simulink model "Quadrotor_two_blocks_v3"  (R2020a)
settings: Solver=FixedStepAuto  StartTime=0.0  StopTime=options.T_train  FixedStep=options.dt  RelTol=1e-6
undefined symbols (not defined in the file or in its folder): options, Quad
libraries: neural x87
(part 3 of 5)

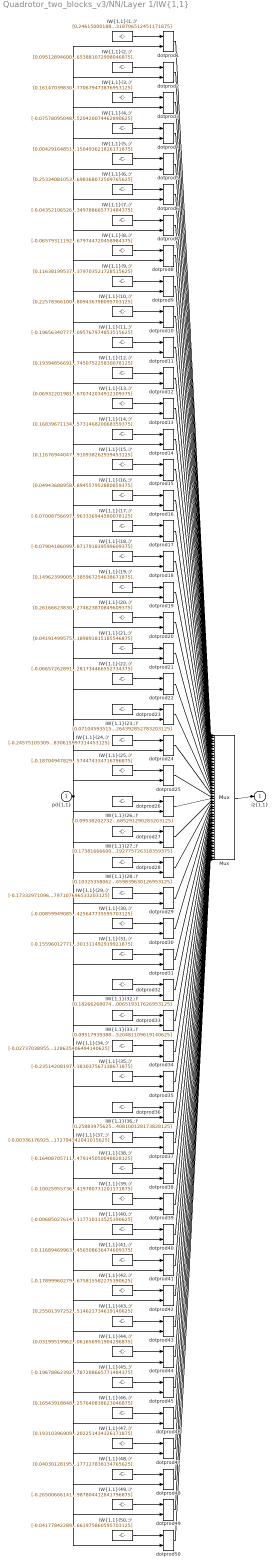
== system Quadrotor_two_blocks_v3/NN/Layer 1/IW{1,1} ==
  "pd{1,1}" : Inport  PortDimensions=15
      mask Display: e = 0.06;c1 = [120 230 180]/255;c2 = ([120 230 180]+0)/(256+128);c3 = ([120 230 180]+128)/(256+128);patch([0 1 1 0],[0 0 1 1],c1);patch([0 1 1 1-e 1-e 0+e],[0 0 1 1-e 0+e 0+e],c2);patch([0 0 1 1-e 0+e 0+e],[0 1 1 1-e 1-e 0+e],c3);plot([0 1 1 0 0],[0 0 1 1 0]);
  "IW{1,1}(1,:)'" : Constant  Value=[0.24615000188350677490234375;-0.2769688665866851806640625;0.19857059419155120849609375;-0.188253819942474365234375;-0.2332561910152435302734375;0.2510521709918975830078125;0.09584285318851470947265625;0.19580931961536407470703125;-0.05497033894062042236328125;-0.1999491155147552490234375;0.0023749410174787044525146484375;-0.1995990574359893798828125;-0.03645892441272735595703125;0.22868992388248443603515625;0.1527912318706512451171875]
      mask Display: e = 0.06;c1 = [120 150 230]/255;c2 = ([120 150 230]+0)/383;c3 = ([120 150 230]+128)/383;patch([0 1 1 0],[0 0 1 1],c1);patch([0 1 1 1-e 1-e 0+e],[0 0 1 1-e 0+e 0+e],c2);patch([0 0 1 1-e 0+e 0+e],[0 1 1 1-e 1-e 0+e],c3);plot([0 1 1 0 0],[0 0 1 1 0]);disp('Weights');
  "IW{1,1}(10,:)'" : Constant  Value=[0.22578366100788116455078125;0.1848590075969696044921875;0.02715091407299041748046875;-0.2515232563018798828125;-0.119150958955287933349609375;-0.2643735110759735107421875;-0.170074880123138427734375;-0.12265492975711822509765625;-0.15844647586345672607421875;-0.035431392490863800048828125;-0.012248366139829158782958984375;0.2504398822784423828125;0.2176316678524017333984375;-0.121464140713214874267578125;0.24602694809436798095703125]
      mask Display: e = 0.06;c1 = [120 150 230]/255;c2 = ([120 150 230]+0)/383;c3 = ([120 150 230]+128)/383;patch([0 1 1 0],[0 0 1 1],c1);patch([0 1 1 1-e 1-e 0+e],[0 0 1 1-e 0+e 0+e],c2);patch([0 0 1 1-e 0+e 0+e],[0 1 1 1-e 1-e 0+e],c3);plot([0 1 1 0 0],[0 0 1 1 0]);disp('Weights');
  "IW{1,1}(11,:)'" : Constant  Value=[-0.19656340777873992919921875;0.19387482106685638427734375;-0.0459356568753719329833984375;0.2647550404071807861328125;0.2745810449123382568359375;0.041675679385662078857421875;0.12391470372676849365234375;-0.16976629197597503662109375;0.0317076109349727630615234375;0.080004759132862091064453125;0.18198011815547943115234375;0.2869862020015716552734375;-0.145103871822357177734375;-0.1056883335113525390625;-0.17829205095767974853515625]
      mask Display: e = 0.06;c1 = [120 150 230]/255;c2 = ([120 150 230]+0)/383;c3 = ([120 150 230]+128)/383;patch([0 1 1 0],[0 0 1 1],c1);patch([0 1 1 1-e 1-e 0+e],[0 0 1 1-e 0+e 0+e],c2);patch([0 0 1 1-e 0+e 0+e],[0 1 1 1-e 1-e 0+e],c3);plot([0 1 1 0 0],[0 0 1 1 0]);disp('Weights');
  "IW{1,1}(12,:)'" : Constant  Value=[0.193948566913604736328125;-0.19000457227230072021484375;-0.086530886590480804443359375;-0.180632650852203369140625;-0.19515524804592132568359375;-0.0314301587641239166259765625;0.1326048672199249267578125;0.2292857468128204345703125;0.13057291507720947265625;-0.196017682552337646484375;-0.267640650272369384765625;0.018295593559741973876953125;0.092189691960811614990234375;0.2637727260589599609375;0.3198082745075225830078125]
      mask Display: e = 0.06;c1 = [120 150 230]/255;c2 = ([120 150 230]+0)/383;c3 = ([120 150 230]+128)/383;patch([0 1 1 0],[0 0 1 1],c1);patch([0 1 1 1-e 1-e 0+e],[0 0 1 1-e 0+e 0+e],c2);patch([0 0 1 1-e 0+e 0+e],[0 1 1 1-e 1-e 0+e],c3);plot([0 1 1 0 0],[0 0 1 1 0]);disp('Weights');
  "IW{1,1}(13,:)'" : Constant  Value=[0.0693220198154449462890625;-0.2461332976818084716796875;-0.0500579774379730224609375;0.154254257678985595703125;0.03849256038665771484375;0.23319505155086517333984375;-0.2198602855205535888671875;0.0940903127193450927734375;0.068703256547451019287109375;0.3237433731555938720703125;0.282208859920501708984375;0.054376460611820220947265625;-0.110324062407016754150390625;-0.195249617099761962890625;0.1259351670742034912109375]
      mask Display: e = 0.06;c1 = [120 150 230]/255;c2 = ([120 150 230]+0)/383;c3 = ([120 150 230]+128)/383;patch([0 1 1 0],[0 0 1 1],c1);patch([0 1 1 1-e 1-e 0+e],[0 0 1 1-e 0+e 0+e],c2);patch([0 0 1 1-e 0+e 0+e],[0 1 1 1-e 1-e 0+e],c3);plot([0 1 1 0 0],[0 0 1 1 0]);disp('Weights');
  "IW{1,1}(14,:)'" : Constant  Value=[0.1683967113494873046875;-0.20133976638317108154296875;-0.0863095223903656005859375;-0.20713274180889129638671875;-0.0525672137737274169921875;0.090336024761199951171875;0.209331095218658447265625;-0.02543685026466846466064453125;-0.2690856456756591796875;-0.12498508393764495849609375;-0.2766831815242767333984375;-0.08764405548572540283203125;-0.082091726362705230712890625;0.0041847997345030307769775390625;0.035477362573146820068359375]
      mask Display: e = 0.06;c1 = [120 150 230]/255;c2 = ([120 150 230]+0)/383;c3 = ([120 150 230]+128)/383;patch([0 1 1 0],[0 0 1 1],c1);patch([0 1 1 1-e 1-e 0+e],[0 0 1 1-e 0+e 0+e],c2);patch([0 0 1 1-e 0+e 0+e],[0 1 1 1-e 1-e 0+e],c3);plot([0 1 1 0 0],[0 0 1 1 0]);disp('Weights');
  "IW{1,1}(15,:)'" : Constant  Value=[0.116769440472126007080078125;0.1042247116565704345703125;0.237415611743927001953125;-0.2428454458713531494140625;0.040846385061740875244140625;-0.13717560470104217529296875;0.063017547130584716796875;-0.13246162235736846923828125;0.262563228607177734375;-0.05162282288074493408203125;-0.076942525804042816162109375;0.0027029174380004405975341796875;-0.069335155189037322998046875;0.075416088104248046875;-0.17622537910938262939453125]
      mask Display: e = 0.06;c1 = [120 150 230]/255;c2 = ([120 150 230]+0)/383;c3 = ([120 150 230]+128)/383;patch([0 1 1 0],[0 0 1 1],c1);patch([0 1 1 1-e 1-e 0+e],[0 0 1 1-e 0+e 0+e],c2);patch([0 0 1 1-e 0+e 0+e],[0 1 1 1-e 1-e 0+e],c3);plot([0 1 1 0 0],[0 0 1 1 0]);disp('Weights');
  "IW{1,1}(16,:)'" : Constant  Value=[0.049436889588832855224609375;0.21147786080837249755859375;-0.14443112909793853759765625;0.014394345693290233612060546875;-0.1196068823337554931640625;0.19549985229969024658203125;0.0031798514537513256072998046875;0.116258658468723297119140625;0.01721403189003467559814453125;-0.01672693900763988494873046875;0.107975371181964874267578125;-0.1965630948543548583984375;-0.0043267779983580112457275390625;0.0615588091313838958740234375;-0.035299263894557952880859375]
      mask Display: e = 0.06;c1 = [120 150 230]/255;c2 = ([120 150 230]+0)/383;c3 = ([120 150 230]+128)/383;patch([0 1 1 0],[0 0 1 1],c1);patch([0 1 1 1-e 1-e 0+e],[0 0 1 1-e 0+e 0+e],c2);patch([0 0 1 1-e 0+e 0+e],[0 1 1 1-e 1-e 0+e],c3);plot([0 1 1 0 0],[0 0 1 1 0]);disp('Weights');
  "IW{1,1}(17,:)'" : Constant  Value=[-0.07008756697177886962890625;0.15847004950046539306640625;0.2939801514148712158203125;-0.224480688571929931640625;-0.21031963825225830078125;-0.13364918529987335205078125;-0.048141755163669586181640625;-0.02383042313158512115478515625;-0.22567288577556610107421875;0.295534789562225341796875;0.18090365827083587646484375;-0.074320316314697265625;-0.2824363410472869873046875;0.25463569164276123046875;-0.2515518963336944580078125]
      mask Display: e = 0.06;c1 = [120 150 230]/255;c2 = ([120 150 230]+0)/383;c3 = ([120 150 230]+128)/383;patch([0 1 1 0],[0 0 1 1],c1);patch([0 1 1 1-e 1-e 0+e],[0 0 1 1-e 0+e 0+e],c2);patch([0 0 1 1-e 0+e 0+e],[0 1 1 1-e 1-e 0+e],c3);plot([0 1 1 0 0],[0 0 1 1 0]);disp('Weights');
  "IW{1,1}(18,:)'" : Constant  Value=[-0.079041860997676849365234375;-0.073680095374584197998046875;0.02200210280716419219970703125;-0.21910385787487030029296875;-0.2514393627643585205078125;-0.055510602891445159912109375;0.069919586181640625;0.2702545225620269775390625;0.21673555672168731689453125;0.24634529650211334228515625;0.058262996375560760498046875;-0.0304315388202667236328125;-0.133230149745941162109375;-0.16089808940887451171875;-0.010348445735871791839599609375]
      mask Display: e = 0.06;c1 = [120 150 230]/255;c2 = ([120 150 230]+0)/383;c3 = ([120 150 230]+128)/383;patch([0 1 1 0],[0 0 1 1],c1);patch([0 1 1 1-e 1-e 0+e],[0 0 1 1-e 0+e 0+e],c2);patch([0 0 1 1-e 0+e 0+e],[0 1 1 1-e 1-e 0+e],c3);plot([0 1 1 0 0],[0 0 1 1 0]);disp('Weights');
  "IW{1,1}(19,:)'" : Constant  Value=[0.14962399005889892578125;-0.16748203337192535400390625;0.14350183308124542236328125;-0.2470430433750152587890625;-0.002806025557219982147216796875;0.1744572222232818603515625;-0.1394075453281402587890625;0.15507133305072784423828125;-0.090710349380970001220703125;0.145454347133636474609375;-0.13279436528682708740234375;0.083461605012416839599609375;-0.0711586773395538330078125;0.0425617434084415435791015625;-0.20231859385967254638671875]
      mask Display: e = 0.06;c1 = [120 150 230]/255;c2 = ([120 150 230]+0)/383;c3 = ([120 150 230]+128)/383;patch([0 1 1 0],[0 0 1 1],c1);patch([0 1 1 1-e 1-e 0+e],[0 0 1 1-e 0+e 0+e],c2);patch([0 0 1 1-e 0+e 0+e],[0 1 1 1-e 1-e 0+e],c3);plot([0 1 1 0 0],[0 0 1 1 0]);disp('Weights');
  "IW{1,1}(2,:)'" : Constant  Value=[0.095128946006298065185546875;-0.22730006277561187744140625;0.1379710733890533447265625;-0.22612141072750091552734375;-0.2971851527690887451171875;-0.0599823035299777984619140625;-0.066525168716907501220703125;0.17862474918365478515625;0.02654240839183330535888671875;0.050377599895000457763671875;-0.14958135783672332763671875;0.076478295028209686279296875;0.0403922982513904571533203125;-0.272404968738555908203125;0.077281653881072998046875]
      mask Display: e = 0.06;c1 = [120 150 230]/255;c2 = ([120 150 230]+0)/383;c3 = ([120 150 230]+128)/383;patch([0 1 1 0],[0 0 1 1],c1);patch([0 1 1 1-e 1-e 0+e],[0 0 1 1-e 0+e 0+e],c2);patch([0 0 1 1-e 0+e 0+e],[0 1 1 1-e 1-e 0+e],c3);plot([0 1 1 0 0],[0 0 1 1 0]);disp('Weights');
  "IW{1,1}(20,:)'" : Constant  Value=[0.261666238307952880859375;0.02036500163376331329345703125;0.25814878940582275390625;0.138574182987213134765625;-0.3060087859630584716796875;0.20479990541934967041015625;0.20900227129459381103515625;0.2794874608516693115234375;0.23982979357242584228515625;-0.2558719217777252197265625;0.16411621868610382080078125;0.23556821048259735107421875;0.014061002992093563079833984375;-0.32590019702911376953125;-0.306461274623870849609375]
      mask Display: e = 0.06;c1 = [120 150 230]/255;c2 = ([120 150 230]+0)/383;c3 = ([120 150 230]+128)/383;patch([0 1 1 0],[0 0 1 1],c1);patch([0 1 1 1-e 1-e 0+e],[0 0 1 1-e 0+e 0+e],c2);patch([0 0 1 1-e 0+e 0+e],[0 1 1 1-e 1-e 0+e],c3);plot([0 1 1 0 0],[0 0 1 1 0]);disp('Weights');
  "IW{1,1}(21,:)'" : Constant  Value=[0.0419149957597255706787109375;-0.1758421361446380615234375;-0.085287906229496002197265625;0.012431069277226924896240234375;0.18711845576763153076171875;-0.20032370090484619140625;-0.118400655686855316162109375;-0.268635094165802001953125;0.19941572844982147216796875;0.01469893567264080047607421875;0.0416434891521930694580078125;0.0564967282116413116455078125;0.121020205318927764892578125;-0.2310643494129180908203125;0.22104959189891815185546875]
      mask Display: e = 0.06;c1 = [120 150 230]/255;c2 = ([120 150 230]+0)/383;c3 = ([120 150 230]+128)/383;patch([0 1 1 0],[0 0 1 1],c1);patch([0 1 1 1-e 1-e 0+e],[0 0 1 1-e 0+e 0+e],c2);patch([0 0 1 1-e 0+e 0+e],[0 1 1 1-e 1-e 0+e],c3);plot([0 1 1 0 0],[0 0 1 1 0]);disp('Weights');
  "IW{1,1}(22,:)'" : Constant  Value=[-0.066572628915309906005859375;-0.20581817626953125;0.2635544240474700927734375;0.12549085915088653564453125;-0.22472874820232391357421875;-0.32307136058807373046875;0.01963965408504009246826171875;-0.2814792096614837646484375;-0.02858440019190311431884765625;0.0336724705994129180908203125;-0.2505728304386138916015625;-0.119029082357883453369140625;0.0365916155278682708740234375;0.24474680423736572265625;-0.051868580281734466552734375]
      mask Display: e = 0.06;c1 = [120 150 230]/255;c2 = ([120 150 230]+0)/383;c3 = ([120 150 230]+128)/383;patch([0 1 1 0],[0 0 1 1],c1);patch([0 1 1 1-e 1-e 0+e],[0 0 1 1-e 0+e 0+e],c2);patch([0 0 1 1-e 0+e 0+e],[0 1 1 1-e 1-e 0+e],c3);plot([0 1 1 0 0],[0 0 1 1 0]);disp('Weights');
  "IW{1,1}(23,:)'" : Constant  Value=[0.071045935153961181640625;-0.21809609234333038330078125;0.05046935379505157470703125;0.069395743310451507568359375;0.0854937136173248291015625;-0.19188939034938812255859375;-0.0527186132967472076416015625;-0.091981507837772369384765625;-0.1890372335910797119140625;-0.1783023178577423095703125;-0.123200200498104095458984375;0.067269988358020782470703125;0.110163219273090362548828125;0.115163743495941162109375;0.0615452714264392852783203125]
      mask Display: e = 0.06;c1 = [120 150 230]/255;c2 = ([120 150 230]+0)/383;c3 = ([120 150 230]+128)/383;patch([0 1 1 0],[0 0 1 1],c1);patch([0 1 1 1-e 1-e 0+e],[0 0 1 1-e 0+e 0+e],c2);patch([0 0 1 1-e 0+e 0+e],[0 1 1 1-e 1-e 0+e],c3);plot([0 1 1 0 0],[0 0 1 1 0]);disp('Weights');
  "IW{1,1}(24,:)'" : Constant  Value=[-0.2457510530948638916015625;-0.00290061696432530879974365234375;0.0628999769687652587890625;-0.0369785390794277191162109375;-0.21306161582469940185546875;-0.11851297318935394287109375;-0.101107947528362274169921875;0.097452946007251739501953125;-0.02273922599852085113525390625;0.1242475807666778564453125;-0.048373006284236907958984375;-0.18220658600330352783203125;0.018271021544933319091796875;0.06626848876476287841796875;0.307836830615997314453125]
      mask Display: e = 0.06;c1 = [120 150 230]/255;c2 = ([120 150 230]+0)/383;c3 = ([120 150 230]+128)/383;patch([0 1 1 0],[0 0 1 1],c1);patch([0 1 1 1-e 1-e 0+e],[0 0 1 1-e 0+e 0+e],c2);patch([0 0 1 1-e 0+e 0+e],[0 1 1 1-e 1-e 0+e],c3);plot([0 1 1 0 0],[0 0 1 1 0]);disp('Weights');
  "IW{1,1}(25,:)'" : Constant  Value=[-0.1870494782924652099609375;0.23432266712188720703125;-0.13851954042911529541015625;0.2862237989902496337890625;0.21341784298419952392578125;0.110001362860202789306640625;0.148874759674072265625;-0.107599027454853057861328125;-0.1939537227153778076171875;-0.2659693658351898193359375;-0.14962039887905120849609375;-0.253358781337738037109375;0.0337832234799861907958984375;-0.011594393290579319000244140625;-0.1259245574474334716796875]
      mask Display: e = 0.06;c1 = [120 150 230]/255;c2 = ([120 150 230]+0)/383;c3 = ([120 150 230]+128)/383;patch([0 1 1 0],[0 0 1 1],c1);patch([0 1 1 1-e 1-e 0+e],[0 0 1 1-e 0+e 0+e],c2);patch([0 0 1 1-e 0+e 0+e],[0 1 1 1-e 1-e 0+e],c3);plot([0 1 1 0 0],[0 0 1 1 0]);disp('Weights');
  "IW{1,1}(26,:)'" : Constant  Value=[-0.095382027328014373779296875;-0.043266214430332183837890625;-0.283170282840728759765625;0.15734611451625823974609375;0.121022947132587432861328125;-0.100933618843555450439453125;0.073748223483562469482421875;-0.1514988243579864501953125;0.076255895197391510009765625;-0.00151985208503901958465576171875;0.23000343143939971923828125;-0.2195928394794464111328125;-0.06195227801799774169921875;-0.3127676546573638916015625;0.0615214295685291290283203125]
      mask Display: e = 0.06;c1 = [120 150 230]/255;c2 = ([120 150 230]+0)/383;c3 = ([120 150 230]+128)/383;patch([0 1 1 0],[0 0 1 1],c1);patch([0 1 1 1-e 1-e 0+e],[0 0 1 1-e 0+e 0+e],c2);patch([0 0 1 1-e 0+e 0+e],[0 1 1 1-e 1-e 0+e],c3);plot([0 1 1 0 0],[0 0 1 1 0]);disp('Weights');
  "IW{1,1}(27,:)'" : Constant  Value=[0.17381666600704193115234375;-0.23211638629436492919921875;0.1268526613712310791015625;0.06865088641643524169921875;-0.17158119380474090576171875;-0.068425603210926055908203125;0.1480681002140045166015625;0.085741259157657623291015625;-0.1382149159908294677734375;-0.117167912423610687255859375;0.2423031330108642578125;0.0059379111044108867645263671875;0.014612124301493167877197265625;0.051668755710124969482421875;0.094148360192775726318359375]
      mask Display: e = 0.06;c1 = [120 150 230]/255;c2 = ([120 150 230]+0)/383;c3 = ([120 150 230]+128)/383;patch([0 1 1 0],[0 0 1 1],c1);patch([0 1 1 1-e 1-e 0+e],[0 0 1 1-e 0+e 0+e],c2);patch([0 0 1 1-e 0+e 0+e],[0 1 1 1-e 1-e 0+e],c3);plot([0 1 1 0 0],[0 0 1 1 0]);disp('Weights');
  "IW{1,1}(28,:)'" : Constant  Value=[0.103253580629825592041015625;0.2518842220306396484375;-0.102763928472995758056640625;-0.1430141031742095947265625;-0.0503221862018108367919921875;-0.05788277089595794677734375;-0.0347949899733066558837890625;0.098910152912139892578125;-0.223344743251800537109375;-0.076313443481922149658203125;0.1774608790874481201171875;0.24388711154460906982421875;0.2079565227031707763671875;-0.2371452152729034423828125;-0.091363258659839630126953125]
      mask Display: e = 0.06;c1 = [120 150 230]/255;c2 = ([120 150 230]+0)/383;c3 = ([120 150 230]+128)/383;patch([0 1 1 0],[0 0 1 1],c1);patch([0 1 1 1-e 1-e 0+e],[0 0 1 1-e 0+e 0+e],c2);patch([0 0 1 1-e 0+e 0+e],[0 1 1 1-e 1-e 0+e],c3);plot([0 1 1 0 0],[0 0 1 1 0]);disp('Weights');
  "IW{1,1}(29,:)'" : Constant  Value=[-0.17332971096038818359375;-0.167443096637725830078125;0.05027113854885101318359375;0.011691217310726642608642578125;0.1646335124969482421875;-0.1333863437175750732421875;-0.14718823134899139404296875;0.12607334554195404052734375;-0.0293374545872211456298828125;0.22605133056640625;-0.2192026078701019287109375;0.097262375056743621826171875;-0.09161897003650665283203125;-0.1386334598064422607421875;-0.0074653667397797107696533203125]
      mask Display: e = 0.06;c1 = [120 150 230]/255;c2 = ([120 150 230]+0)/383;c3 = ([120 150 230]+128)/383;patch([0 1 1 0],[0 0 1 1],c1);patch([0 1 1 1-e 1-e 0+e],[0 0 1 1-e 0+e 0+e],c2);patch([0 0 1 1-e 0+e 0+e],[0 1 1 1-e 1-e 0+e],c3);plot([0 1 1 0 0],[0 0 1 1 0]);disp('Weights');
  "IW{1,1}(3,:)'" : Constant  Value=[0.16147039830684661865234375;0.21830980479717254638671875;-0.17483437061309814453125;-0.081198640167713165283203125;-0.13683383166790008544921875;0.0219206102192401885986328125;-0.044701538980007171630859375;-0.00686088390648365020751953125;-0.16412331163883209228515625;-0.0458278357982635498046875;-0.0192497037351131439208984375;0.00805437564849853515625;0.099379234015941619873046875;0.3053427636623382568359375;0.01863983459770679473876953125]
      mask Display: e = 0.06;c1 = [120 150 230]/255;c2 = ([120 150 230]+0)/383;c3 = ([120 150 230]+128)/383;patch([0 1 1 0],[0 0 1 1],c1);patch([0 1 1 1-e 1-e 0+e],[0 0 1 1-e 0+e 0+e],c2);patch([0 0 1 1-e 0+e 0+e],[0 1 1 1-e 1-e 0+e],c3);plot([0 1 1 0 0],[0 0 1 1 0]);disp('Weights');
  "IW{1,1}(30,:)'" : Constant  Value=[-0.008599490858614444732666015625;-0.097333796322345733642578125;-0.076125584542751312255859375;-0.2967312335968017578125;-0.0456822775304317474365234375;0.1023000180721282958984375;-0.22809056937694549560546875;-0.18679632246494293212890625;-0.23915708065032958984375;0.21873106062412261962890625;-0.2036375701427459716796875;0.17065073549747467041015625;-0.041879303753376007080078125;-0.083800770342350006103515625;0.2975726425647735595703125]
      mask Display: e = 0.06;c1 = [120 150 230]/255;c2 = ([120 150 230]+0)/383;c3 = ([120 150 230]+128)/383;patch([0 1 1 0],[0 0 1 1],c1);patch([0 1 1 1-e 1-e 0+e],[0 0 1 1-e 0+e 0+e],c2);patch([0 0 1 1-e 0+e 0+e],[0 1 1 1-e 1-e 0+e],c3);plot([0 1 1 0 0],[0 0 1 1 0]);disp('Weights');
  "IW{1,1}(31,:)'" : Constant  Value=[-0.15596012771129608154296875;-0.23804713785648345947265625;-0.09500749409198760986328125;-0.197879850864410400390625;0.21830274164676666259765625;0.200557410717010498046875;0.101521052420139312744140625;0.07105290889739990234375;0.083333194255828857421875;-0.09866882860660552978515625;-0.10722625255584716796875;-0.271394908428192138671875;-0.02957780472934246063232421875;0.100286401808261871337890625;0.1091277301311492919921875]
      mask Display: e = 0.06;c1 = [120 150 230]/255;c2 = ([120 150 230]+0)/383;c3 = ([120 150 230]+128)/383;patch([0 1 1 0],[0 0 1 1],c1);patch([0 1 1 1-e 1-e 0+e],[0 0 1 1-e 0+e 0+e],c2);patch([0 0 1 1-e 0+e 0+e],[0 1 1 1-e 1-e 0+e],c3);plot([0 1 1 0 0],[0 0 1 1 0]);disp('Weights');
  "IW{1,1}(32,:)'" : Constant  Value=[0.18266268074512481689453125;0.052521593868732452392578125;-0.2643826007843017578125;0.02975536696612834930419921875;-0.0076476526446640491485595703125;-0.0893814563751220703125;-0.20603883266448974609375;-0.342833697795867919921875;0.1492862701416015625;0.07950533926486968994140625;-0.0254016630351543426513671875;-0.0215784944593906402587890625;0.1966168582439422607421875;0.2676563560962677001953125;0.23761864006519317626953125]
      mask Display: e = 0.06;c1 = [120 150 230]/255;c2 = ([120 150 230]+0)/383;c3 = ([120 150 230]+128)/383;patch([0 1 1 0],[0 0 1 1],c1);patch([0 1 1 1-e 1-e 0+e],[0 0 1 1-e 0+e 0+e],c2);patch([0 0 1 1-e 0+e 0+e],[0 1 1 1-e 1-e 0+e],c3);plot([0 1 1 0 0],[0 0 1 1 0]);disp('Weights');
  "IW{1,1}(33,:)'" : Constant  Value=[0.09517939388751983642578125;0.15935568511486053466796875;0.21380753815174102783203125;0.22671794891357421875;-0.07564093172550201416015625;-0.12772651016712188720703125;0.132677972316741943359375;-0.15164233744144439697265625;-0.09782598912715911865234375;-0.184073030948638916015625;0.21864677965641021728515625;-0.152646243572235107421875;-0.0016746222972869873046875;-0.02401728741824626922607421875;-0.15558661520481109619140625]
      mask Display: e = 0.06;c1 = [120 150 230]/255;c2 = ([120 150 230]+0)/383;c3 = ([120 150 230]+128)/383;patch([0 1 1 0],[0 0 1 1],c1);patch([0 1 1 1-e 1-e 0+e],[0 0 1 1-e 0+e 0+e],c2);patch([0 0 1 1-e 0+e 0+e],[0 1 1 1-e 1-e 0+e],c3);plot([0 1 1 0 0],[0 0 1 1 0]);disp('Weights');
  "IW{1,1}(34,:)'" : Constant  Value=[-0.0273703895509243011474609375;-0.229876697063446044921875;0.20097278058528900146484375;0.07791368663311004638671875;0.0347439944744110107421875;-0.19273804128170013427734375;0.0321986861526966094970703125;0.113342873752117156982421875;0.087004609405994415283203125;-0.1804614961147308349609375;0.12650966644287109375;0.168824613094329833984375;0.051381371915340423583984375;-0.313193798065185546875;0.00304802157916128635406494140625]
      mask Display: e = 0.06;c1 = [120 150 230]/255;c2 = ([120 150 230]+0)/383;c3 = ([120 150 230]+128)/383;patch([0 1 1 0],[0 0 1 1],c1);patch([0 1 1 1-e 1-e 0+e],[0 0 1 1-e 0+e 0+e],c2);patch([0 0 1 1-e 0+e 0+e],[0 1 1 1-e 1-e 0+e],c3);plot([0 1 1 0 0],[0 0 1 1 0]);disp('Weights');
  "IW{1,1}(35,:)'" : Constant  Value=[-0.2351420819759368896484375;0.2611202895641326904296875;-0.076084636151790618896484375;-0.3368081748485565185546875;-0.146379947662353515625;0.096819393336772918701171875;-0.089184351265430450439453125;0.1102201938629150390625;-0.06919331848621368408203125;-0.16959495842456817626953125;-0.121027551591396331787109375;-0.0278002656996250152587890625;0.1924916207790374755859375;-0.15046937763690948486328125;0.1281383037567138671875]
      mask Display: e = 0.06;c1 = [120 150 230]/255;c2 = ([120 150 230]+0)/383;c3 = ([120 150 230]+128)/383;patch([0 1 1 0],[0 0 1 1],c1);patch([0 1 1 1-e 1-e 0+e],[0 0 1 1-e 0+e 0+e],c2);patch([0 0 1 1-e 0+e 0+e],[0 1 1 1-e 1-e 0+e],c3);plot([0 1 1 0 0],[0 0 1 1 0]);disp('Weights');
  "IW{1,1}(36,:)'" : Constant  Value=[0.2588397562503814697265625;-0.058032773435115814208984375;0.111643381416797637939453125;0.092710889875888824462890625;0.0520550496876239776611328125;0.03596360981464385986328125;0.0407148301601409912109375;-0.11636646091938018798828125;-0.1568354666233062744140625;0.22985266149044036865234375;-0.0419293679296970367431640625;-0.227225720882415771484375;-0.222439348697662353515625;-0.2294310629367828369140625;0.16932876408100128173828125]
      mask Display: e = 0.06;c1 = [120 150 230]/255;c2 = ([120 150 230]+0)/383;c3 = ([120 150 230]+128)/383;patch([0 1 1 0],[0 0 1 1],c1);patch([0 1 1 1-e 1-e 0+e],[0 0 1 1-e 0+e 0+e],c2);patch([0 0 1 1-e 0+e 0+e],[0 1 1 1-e 1-e 0+e],c3);plot([0 1 1 0 0],[0 0 1 1 0]);disp('Weights');
  "IW{1,1}(37,:)'" : Constant  Value=[-0.00336176925338804721832275390625;-0.096880234777927398681640625;0.01142371632158756256103515625;0.16033767163753509521484375;-0.168270111083984375;0.1665506064891815185546875;0.0410696230828762054443359375;0.140136778354644775390625;0.17146994173526763916015625;-0.072415925562381744384765625;-0.05427610874176025390625;0.2096602022647857666015625;0.0733962357044219970703125;-0.08000452816486358642578125;-0.062596537172794342041015625]
      mask Display: e = 0.06;c1 = [120 150 230]/255;c2 = ([120 150 230]+0)/383;c3 = ([120 150 230]+128)/383;patch([0 1 1 0],[0 0 1 1],c1);patch([0 1 1 1-e 1-e 0+e],[0 0 1 1-e 0+e 0+e],c2);patch([0 0 1 1-e 0+e 0+e],[0 1 1 1-e 1-e 0+e],c3);plot([0 1 1 0 0],[0 0 1 1 0]);disp('Weights');
  "IW{1,1}(38,:)'" : Constant  Value=[-0.1640870571136474609375;0.1660376489162445068359375;0.010183542035520076751708984375;-0.01128961704671382904052734375;0.24906851351261138916015625;0.0410409159958362579345703125;0.13058064877986907958984375;0.0533278845250606536865234375;-0.0908943116664886474609375;-0.227045834064483642578125;0.333160400390625;0.264751613140106201171875;0.0366494245827198028564453125;-0.1303275525569915771484375;-0.14577205479145050048828125]
      mask Display: e = 0.06;c1 = [120 150 230]/255;c2 = ([120 150 230]+0)/383;c3 = ([120 150 230]+128)/383;patch([0 1 1 0],[0 0 1 1],c1);patch([0 1 1 1-e 1-e 0+e],[0 0 1 1-e 0+e 0+e],c2);patch([0 0 1 1-e 0+e 0+e],[0 1 1 1-e 1-e 0+e],c3);plot([0 1 1 0 0],[0 0 1 1 0]);disp('Weights');
  "IW{1,1}(39,:)'" : Constant  Value=[-0.10025955736637115478515625;-0.20866437256336212158203125;0.13629941642284393310546875;-0.20547635853290557861328125;0.248189985752105712890625;-0.0040882104076445102691650390625;0.1303304135799407958984375;0.11142595112323760986328125;-0.14620433747768402099609375;-0.0834198892116546630859375;0.194162070751190185546875;0.28933703899383544921875;0.0058604665100574493408203125;0.110569812357425689697265625;-0.1912853419780731201171875]
      mask Display: e = 0.06;c1 = [120 150 230]/255;c2 = ([120 150 230]+0)/383;c3 = ([120 150 230]+128)/383;patch([0 1 1 0],[0 0 1 1],c1);patch([0 1 1 1-e 1-e 0+e],[0 0 1 1-e 0+e 0+e],c2);patch([0 0 1 1-e 0+e 0+e],[0 1 1 1-e 1-e 0+e],c3);plot([0 1 1 0 0],[0 0 1 1 0]);disp('Weights');
  "IW{1,1}(4,:)'" : Constant  Value=[-0.075780950486660003662109375;-0.2693147957324981689453125;0.02768449485301971435546875;-0.02743869833648204803466796875;0.08174251019954681396484375;-0.1477746069431304931640625;0.09734113514423370361328125;-0.08310799300670623779296875;-0.16650156676769256591796875;0.0094405896961688995361328125;-0.09776784479618072509765625;-0.0246720053255558013916015625;-0.036737494170665740966796875;-0.254119575023651123046875;0.0067681097425520420074462890625]
      mask Display: e = 0.06;c1 = [120 150 230]/255;c2 = ([120 150 230]+0)/383;c3 = ([120 150 230]+128)/383;patch([0 1 1 0],[0 0 1 1],c1);patch([0 1 1 1-e 1-e 0+e],[0 0 1 1-e 0+e 0+e],c2);patch([0 0 1 1-e 0+e 0+e],[0 1 1 1-e 1-e 0+e],c3);plot([0 1 1 0 0],[0 0 1 1 0]);disp('Weights');
  "IW{1,1}(40,:)'" : Constant  Value=[-0.0068502761423587799072265625;-0.294479906558990478515625;0.23259864747524261474609375;0.07743291556835174560546875;0.12861360609531402587890625;-0.087664954364299774169921875;-0.14403773844242095947265625;0.097400121390819549560546875;0.19112212955951690673828125;-0.14740465581417083740234375;-0.11749677360057830810546875;-0.1845638751983642578125;0.22564940154552459716796875;0.1084671318531036376953125;0.268547117710113525390625]
      mask Display: e = 0.06;c1 = [120 150 230]/255;c2 = ([120 150 230]+0)/383;c3 = ([120 150 230]+128)/383;patch([0 1 1 0],[0 0 1 1],c1);patch([0 1 1 1-e 1-e 0+e],[0 0 1 1-e 0+e 0+e],c2);patch([0 0 1 1-e 0+e 0+e],[0 1 1 1-e 1-e 0+e],c3);plot([0 1 1 0 0],[0 0 1 1 0]);disp('Weights');
  "IW{1,1}(41,:)'" : Constant  Value=[-0.116894699633121490478515625;0.05900453031063079833984375;-0.0073839430697262287139892578125;0.113214604556560516357421875;0.16053998470306396484375;-0.15438972413539886474609375;0.0062161632813513278961181640625;0.3329826891422271728515625;-0.15763862431049346923828125;-0.16348753869533538818359375;-0.07267363369464874267578125;0.28793585300445556640625;0.109639294445514678955078125;-0.13896895945072174072265625;-0.1695991456508636474609375]
      mask Display: e = 0.06;c1 = [120 150 230]/255;c2 = ([120 150 230]+0)/383;c3 = ([120 150 230]+128)/383;patch([0 1 1 0],[0 0 1 1],c1);patch([0 1 1 1-e 1-e 0+e],[0 0 1 1-e 0+e 0+e],c2);patch([0 0 1 1-e 0+e 0+e],[0 1 1 1-e 1-e 0+e],c3);plot([0 1 1 0 0],[0 0 1 1 0]);disp('Weights');
  "IW{1,1}(42,:)'" : Constant  Value=[-0.178999602794647216796875;-0.273447513580322265625;-0.12310923635959625244140625;0.00014629098586738109588623046875;-0.161006510257720947265625;0.1536577641963958740234375;-0.0535728298127651214599609375;-0.14856360852718353271484375;0.019722230732440948486328125;0.111764647066593170166015625;-0.0299544595181941986083984375;0.13094948232173919677734375;-0.075086347758769989013671875;0.08260428905487060546875;-0.2763656675815582275390625]
      mask Display: e = 0.06;c1 = [120 150 230]/255;c2 = ([120 150 230]+0)/383;c3 = ([120 150 230]+128)/383;patch([0 1 1 0],[0 0 1 1],c1);patch([0 1 1 1-e 1-e 0+e],[0 0 1 1-e 0+e 0+e],c2);patch([0 0 1 1-e 0+e 0+e],[0 1 1 1-e 1-e 0+e],c3);plot([0 1 1 0 0],[0 0 1 1 0]);disp('Weights');
  "IW{1,1}(43,:)'" : Constant  Value=[0.2550139725208282470703125;0.087202854454517364501953125;0.1281315386295318603515625;0.23083533346652984619140625;-0.21401344239711761474609375;0.184855759143829345703125;-0.08882246911525726318359375;0.2115586102008819580078125;-0.16994492709636688232421875;0.02501332946121692657470703125;-0.12911760807037353515625;0.20374305546283721923828125;0.123287834227085113525390625;-0.11168043315410614013671875;-0.08061255514621734619140625]
      mask Display: e = 0.06;c1 = [120 150 230]/255;c2 = ([120 150 230]+0)/383;c3 = ([120 150 230]+128)/383;patch([0 1 1 0],[0 0 1 1],c1);patch([0 1 1 1-e 1-e 0+e],[0 0 1 1-e 0+e 0+e],c2);patch([0 0 1 1-e 0+e 0+e],[0 1 1 1-e 1-e 0+e],c3);plot([0 1 1 0 0],[0 0 1 1 0]);disp('Weights');
  "IW{1,1}(44,:)'" : Constant  Value=[0.031995199620723724365234375;-0.2445659637451171875;0.09365718066692352294921875;-0.01359014213085174560546875;0.115253932774066925048828125;0.193809449672698974609375;0.20953238010406494140625;-0.21192280948162078857421875;0.2081687152385711669921875;0.08719007670879364013671875;0.09894512593746185302734375;-0.3323518931865692138671875;-0.17291621863842010498046875;-0.20534498989582061767578125;0.21001248061656951904296875]
      mask Display: e = 0.06;c1 = [120 150 230]/255;c2 = ([120 150 230]+0)/383;c3 = ([120 150 230]+128)/383;patch([0 1 1 0],[0 0 1 1],c1);patch([0 1 1 1-e 1-e 0+e],[0 0 1 1-e 0+e 0+e],c2);patch([0 0 1 1-e 0+e 0+e],[0 1 1 1-e 1-e 0+e],c3);plot([0 1 1 0 0],[0 0 1 1 0]);disp('Weights');
  "IW{1,1}(45,:)'" : Constant  Value=[-0.19678862392902374267578125;0.2786497175693511962890625;-0.23901598155498504638671875;0.08081722259521484375;-0.160028398036956787109375;0.0243616290390491485595703125;-0.16942380368709564208984375;0.18367920815944671630859375;0.18878172338008880615234375;0.13933406770229339599609375;-0.089591898024082183837890625;-0.1950030028820037841796875;0.0060748434625566005706787109375;-0.1838549673557281494140625;-0.161368787288665771484375]
      mask Display: e = 0.06;c1 = [120 150 230]/255;c2 = ([120 150 230]+0)/383;c3 = ([120 150 230]+128)/383;patch([0 1 1 0],[0 0 1 1],c1);patch([0 1 1 1-e 1-e 0+e],[0 0 1 1-e 0+e 0+e],c2);patch([0 0 1 1-e 0+e 0+e],[0 1 1 1-e 1-e 0+e],c3);plot([0 1 1 0 0],[0 0 1 1 0]);disp('Weights');
  "IW{1,1}(46,:)'" : Constant  Value=[0.165439188480377197265625;-0.0480287969112396240234375;0.09643124043941497802734375;-0.250464737415313720703125;0.12535963952541351318359375;0.25729274749755859375;-0.0290462486445903778076171875;0.09611950814723968505859375;-0.032192014157772064208984375;0.15565316379070281982421875;0.2400987148284912109375;0.063754625618457794189453125;-0.109129764139652252197265625;-0.16248153150081634521484375;-0.15873794257640838623046875]
      mask Display: e = 0.06;c1 = [120 150 230]/255;c2 = ([120 150 230]+0)/383;c3 = ([120 150 230]+128)/383;patch([0 1 1 0],[0 0 1 1],c1);patch([0 1 1 1-e 1-e 0+e],[0 0 1 1-e 0+e 0+e],c2);patch([0 0 1 1-e 0+e 0+e],[0 1 1 1-e 1-e 0+e],c3);plot([0 1 1 0 0],[0 0 1 1 0]);disp('Weights');
  "IW{1,1}(47,:)'" : Constant  Value=[0.193103969097137451171875;0.281725347042083740234375;-0.123319685459136962890625;-0.0739574134349822998046875;0.07788087427616119384765625;0.2269176542758941650390625;-0.0030886717140674591064453125;-0.2560182511806488037109375;0.13915073871612548828125;0.0589893423020839691162109375;-0.115796267986297607421875;-0.2455928325653076171875;-0.15703094005584716796875;-0.09021453559398651123046875;-0.044255249202251434326171875]
      mask Display: e = 0.06;c1 = [120 150 230]/255;c2 = ([120 150 230]+0)/383;c3 = ([120 150 230]+128)/383;patch([0 1 1 0],[0 0 1 1],c1);patch([0 1 1 1-e 1-e 0+e],[0 0 1 1-e 0+e 0+e],c2);patch([0 0 1 1-e 0+e 0+e],[0 1 1 1-e 1-e 0+e],c3);plot([0 1 1 0 0],[0 0 1 1 0]);disp('Weights');
  "IW{1,1}(48,:)'" : Constant  Value=[0.0403012819588184356689453125;0.0427220799028873443603515625;-0.17625553905963897705078125;-0.2082243263721466064453125;-0.102192573249340057373046875;0.05307517945766448974609375;-0.0062423082999885082244873046875;-0.07624222338199615478515625;0.0435219593346118927001953125;0.15924017131328582763671875;-0.056298308074474334716796875;-0.20113861560821533203125;-0.13641925156116485595703125;-0.23934058845043182373046875;0.00103692547418177127838134765625]
      mask Display: e = 0.06;c1 = [120 150 230]/255;c2 = ([120 150 230]+0)/383;c3 = ([120 150 230]+128)/383;patch([0 1 1 0],[0 0 1 1],c1);patch([0 1 1 1-e 1-e 0+e],[0 0 1 1-e 0+e 0+e],c2);patch([0 0 1 1-e 0+e 0+e],[0 1 1 1-e 1-e 0+e],c3);plot([0 1 1 0 0],[0 0 1 1 0]);disp('Weights');
  "IW{1,1}(49,:)'" : Constant  Value=[-0.26500666141510009765625;0.0445459894835948944091796875;-0.23984424769878387451171875;-0.00298027507960796356201171875;-0.09112976491451263427734375;0.150021612644195556640625;0.01149496994912624359130859375;0.1333840787410736083984375;0.127000749111175537109375;-0.1569814383983612060546875;-0.014628258533775806427001953125;-0.2930984795093536376953125;0.08025334775447845458984375;0.279445171356201171875;0.1811937987804412841796875]
      mask Display: e = 0.06;c1 = [120 150 230]/255;c2 = ([120 150 230]+0)/383;c3 = ([120 150 230]+128)/383;patch([0 1 1 0],[0 0 1 1],c1);patch([0 1 1 1-e 1-e 0+e],[0 0 1 1-e 0+e 0+e],c2);patch([0 0 1 1-e 0+e 0+e],[0 1 1 1-e 1-e 0+e],c3);plot([0 1 1 0 0],[0 0 1 1 0]);disp('Weights');
  "IW{1,1}(5,:)'" : Constant  Value=[0.0042916485108435153961181640625;0.06242644786834716796875;0.08034940063953399658203125;-0.145375430583953857421875;-0.071572028100490570068359375;0.00983425788581371307373046875;0.0300172455608844757080078125;0.1584269702434539794921875;0.278678417205810546875;0.0407252050936222076416015625;0.168755233287811279296875;-0.30025577545166015625;-0.007761939428746700286865234375;0.0387428961694240570068359375;0.20736496150493621826171875]
      mask Display: e = 0.06;c1 = [120 150 230]/255;c2 = ([120 150 230]+0)/383;c3 = ([120 150 230]+128)/383;patch([0 1 1 0],[0 0 1 1],c1);patch([0 1 1 1-e 1-e 0+e],[0 0 1 1-e 0+e 0+e],c2);patch([0 0 1 1-e 0+e 0+e],[0 1 1 1-e 1-e 0+e],c3);plot([0 1 1 0 0],[0 0 1 1 0]);disp('Weights');
  "IW{1,1}(50,:)'" : Constant  Value=[-0.041778422892093658447265625;-0.22763647139072418212890625;-0.0368074215948581695556640625;-0.22750246524810791015625;-0.11225812137126922607421875;0.0162683762609958648681640625;-0.10611288249492645263671875;-0.15786342322826385498046875;0.22624076902866363525390625;-0.146637976169586181640625;0.12673653662204742431640625;-0.07076601684093475341796875;0.103823252022266387939453125;-0.04899288713932037353515625;0.035787768661975860595703125]
      mask Display: e = 0.06;c1 = [120 150 230]/255;c2 = ([120 150 230]+0)/383;c3 = ([120 150 230]+128)/383;patch([0 1 1 0],[0 0 1 1],c1);patch([0 1 1 1-e 1-e 0+e],[0 0 1 1-e 0+e 0+e],c2);patch([0 0 1 1-e 0+e 0+e],[0 1 1 1-e 1-e 0+e],c3);plot([0 1 1 0 0],[0 0 1 1 0]);disp('Weights');
  "IW{1,1}(6,:)'" : Constant  Value=[0.2533408105373382568359375;-0.0433536283671855926513671875;-0.14325940608978271484375;0.20643879473209381103515625;-0.107363045215606689453125;-0.00999970175325870513916015625;-0.090212054550647735595703125;0.03026670776307582855224609375;0.17423152923583984375;0.133468568325042724609375;-0.114795424044132232666015625;-0.0696577727794647216796875;0.0505906827747821807861328125;-0.046158216893672943115234375;0.01735643483698368072509765625]
      mask Display: e = 0.06;c1 = [120 150 230]/255;c2 = ([120 150 230]+0)/383;c3 = ([120 150 230]+128)/383;patch([0 1 1 0],[0 0 1 1],c1);patch([0 1 1 1-e 1-e 0+e],[0 0 1 1-e 0+e 0+e],c2);patch([0 0 1 1-e 0+e 0+e],[0 1 1 1-e 1-e 0+e],c3);plot([0 1 1 0 0],[0 0 1 1 0]);disp('Weights');
  "IW{1,1}(7,:)'" : Constant  Value=[-0.0435210652649402618408203125;0.1514494419097900390625;-0.2734265625476837158203125;0.27500903606414794921875;-0.1378916800022125244140625;0.1153492629528045654296875;-0.0580973513424396514892578125;-0.247794687747955322265625;-0.00294521567411720752716064453125;0.2550494968891143798828125;0.22134526073932647705078125;-0.2774786055088043212890625;-0.156901836395263671875;-0.172052800655364990234375;0.0032655834220349788665771484375]
      mask Display: e = 0.06;c1 = [120 150 230]/255;c2 = ([120 150 230]+0)/383;c3 = ([120 150 230]+128)/383;patch([0 1 1 0],[0 0 1 1],c1);patch([0 1 1 1-e 1-e 0+e],[0 0 1 1-e 0+e 0+e],c2);patch([0 0 1 1-e 0+e 0+e],[0 1 1 1-e 1-e 0+e],c3);plot([0 1 1 0 0],[0 0 1 1 0]);disp('Weights');
  "IW{1,1}(8,:)'" : Constant  Value=[-0.06579311192035675048828125;0.00296015478670597076416015625;-0.186059296131134033203125;0.16186439990997314453125;0.0365433990955352783203125;-0.0924852192401885986328125;0.20830731093883514404296875;0.22138626873493194580078125;0.224468290805816650390625;-0.00245943595655262470245361328125;-0.115652382373809814453125;-0.2189749777317047119140625;-0.010296734981238842010498046875;0.2056125700473785400390625;-0.09135411679744720458984375]
      mask Display: e = 0.06;c1 = [120 150 230]/255;c2 = ([120 150 230]+0)/383;c3 = ([120 150 230]+128)/383;patch([0 1 1 0],[0 0 1 1],c1);patch([0 1 1 1-e 1-e 0+e],[0 0 1 1-e 0+e 0+e],c2);patch([0 0 1 1-e 0+e 0+e],[0 1 1 1-e 1-e 0+e],c3);plot([0 1 1 0 0],[0 0 1 1 0]);disp('Weights');
  "IW{1,1}(9,:)'" : Constant  Value=[0.116381995379924774169921875;0.2902459800243377685546875;-0.2536211311817169189453125;-0.0184618718922138214111328125;-0.19022761285305023193359375;0.03935016691684722900390625;-0.073365949094295501708984375;0.17510007321834564208984375;0.07447980344295501708984375;-0.10619343817234039306640625;0.11082637310028076171875;-0.25694143772125244140625;0.19288730621337890625;0.096076719462871551513671875;-0.27202379703521728515625]
      mask Display: e = 0.06;c1 = [120 150 230]/255;c2 = ([120 150 230]+0)/383;c3 = ([120 150 230]+128)/383;patch([0 1 1 0],[0 0 1 1],c1);patch([0 1 1 1-e 1-e 0+e],[0 0 1 1-e 0+e 0+e],c2);patch([0 0 1 1-e 0+e 0+e],[0 1 1 1-e 1-e 0+e],c3);plot([0 1 1 0 0],[0 0 1 1 0]);disp('Weights');
  Mux : Mux  Inputs=50
      mask Display: e = 0.06;c1 = [120 150 230]/255;c2 = ([120 150 230]+0)/383;c3 = ([120 150 230]+128)/383;patch([0 1 1 0],[0 0 1 1],c1);patch([0 1 1 1-e 1-e 0+e],[0 0 1 1-e 0+e 0+e],c2);patch([0 0 1 1-e 0+e 0+e],[0 1 1 1-e 1-e 0+e],c3);plot([0 1 1 0 0],[0 0 1 1 0]);disp('Mux');
  dotprod{1..50} (50 alike) : neural/Weight Functions/dotprod
  "iz{1,1}" : Outport
      mask Display: e = 0.06;c1 = [120 230 180]/255;c2 = ([120 230 180]+0)/(256+128);c3 = ([120 230 180]+128)/(256+128);patch([0 1 1 0],[0 0 1 1],c1);patch([0 1 1 1-e 1-e 0+e],[0 0 1 1-e 0+e 0+e],c2);patch([0 0 1 1-e 0+e 0+e],[0 1 1 1-e 1-e 0+e],c3);plot([0 1 1 0 0],[0 0 1 1 0]);
  wires:
  "IW{1,1}(1,:)'"/1 -> dotprod1/1
  "pd{1,1}"/1 -> dotprod1/2, dotprod2/2, dotprod3/2, dotprod4/2, dotprod5/2, dotprod6/2, dotprod7/2, dotprod8/2, dotprod9/2, dotprod10/2, dotprod11/2, dotprod12/2, dotprod13/2, dotprod14/2, dotprod15/2, dotprod16/2, dotprod17/2, dotprod18/2, dotprod19/2, dotprod20/2, dotprod21/2, dotprod22/2, dotprod23/2, dotprod24/2, dotprod25/2, dotprod26/2, dotprod27/2, dotprod28/2, dotprod29/2, dotprod30/2, dotprod31/2, dotprod32/2, dotprod33/2, dotprod34/2, dotprod35/2, dotprod36/2, dotprod37/2, dotprod38/2, dotprod39/2, dotprod40/2, dotprod41/2, dotprod42/2, dotprod43/2, dotprod44/2, dotprod45/2, dotprod46/2, dotprod47/2, dotprod48/2, dotprod49/2, dotprod50/2
  dotprod1/1 -> Mux/1
  "IW{1,1}(2,:)'"/1 -> dotprod2/1
  dotprod2/1 -> Mux/2
  "IW{1,1}(3,:)'"/1 -> dotprod3/1
  dotprod3/1 -> Mux/3
  "IW{1,1}(4,:)'"/1 -> dotprod4/1
  dotprod4/1 -> Mux/4
  "IW{1,1}(5,:)'"/1 -> dotprod5/1
  dotprod5/1 -> Mux/5
  "IW{1,1}(6,:)'"/1 -> dotprod6/1
  dotprod6/1 -> Mux/6
  "IW{1,1}(7,:)'"/1 -> dotprod7/1
  dotprod7/1 -> Mux/7
  "IW{1,1}(8,:)'"/1 -> dotprod8/1
  dotprod8/1 -> Mux/8
  "IW{1,1}(9,:)'"/1 -> dotprod9/1
  dotprod9/1 -> Mux/9
  "IW{1,1}(10,:)'"/1 -> dotprod10/1
  dotprod10/1 -> Mux/10
  "IW{1,1}(11,:)'"/1 -> dotprod11/1
  dotprod11/1 -> Mux/11
  "IW{1,1}(12,:)'"/1 -> dotprod12/1
  dotprod12/1 -> Mux/12
  "IW{1,1}(13,:)'"/1 -> dotprod13/1
  dotprod13/1 -> Mux/13
  "IW{1,1}(14,:)'"/1 -> dotprod14/1
  dotprod14/1 -> Mux/14
  "IW{1,1}(15,:)'"/1 -> dotprod15/1
  dotprod15/1 -> Mux/15
  "IW{1,1}(16,:)'"/1 -> dotprod16/1
  dotprod16/1 -> Mux/16
  "IW{1,1}(17,:)'"/1 -> dotprod17/1
  dotprod17/1 -> Mux/17
  "IW{1,1}(18,:)'"/1 -> dotprod18/1
  dotprod18/1 -> Mux/18
  "IW{1,1}(19,:)'"/1 -> dotprod19/1
  dotprod19/1 -> Mux/19
  "IW{1,1}(20,:)'"/1 -> dotprod20/1
  dotprod20/1 -> Mux/20
  "IW{1,1}(21,:)'"/1 -> dotprod21/1
  dotprod21/1 -> Mux/21
  "IW{1,1}(22,:)'"/1 -> dotprod22/1
  dotprod22/1 -> Mux/22
  "IW{1,1}(23,:)'"/1 -> dotprod23/1
  dotprod23/1 -> Mux/23
  "IW{1,1}(24,:)'"/1 -> dotprod24/1
  dotprod24/1 -> Mux/24
  "IW{1,1}(25,:)'"/1 -> dotprod25/1
  dotprod25/1 -> Mux/25
  "IW{1,1}(26,:)'"/1 -> dotprod26/1
  dotprod26/1 -> Mux/26
  "IW{1,1}(27,:)'"/1 -> dotprod27/1
  dotprod27/1 -> Mux/27
  "IW{1,1}(28,:)'"/1 -> dotprod28/1
  dotprod28/1 -> Mux/28
  "IW{1,1}(29,:)'"/1 -> dotprod29/1
  dotprod29/1 -> Mux/29
  "IW{1,1}(30,:)'"/1 -> dotprod30/1
  dotprod30/1 -> Mux/30
  "IW{1,1}(31,:)'"/1 -> dotprod31/1
  dotprod31/1 -> Mux/31
  "IW{1,1}(32,:)'"/1 -> dotprod32/1
  dotprod32/1 -> Mux/32
  "IW{1,1}(33,:)'"/1 -> dotprod33/1
  dotprod33/1 -> Mux/33
  "IW{1,1}(34,:)'"/1 -> dotprod34/1
  dotprod34/1 -> Mux/34
  "IW{1,1}(35,:)'"/1 -> dotprod35/1
  dotprod35/1 -> Mux/35
  "IW{1,1}(36,:)'"/1 -> dotprod36/1
  dotprod36/1 -> Mux/36
  "IW{1,1}(37,:)'"/1 -> dotprod37/1
  dotprod37/1 -> Mux/37
  "IW{1,1}(38,:)'"/1 -> dotprod38/1
  dotprod38/1 -> Mux/38
  "IW{1,1}(39,:)'"/1 -> dotprod39/1
  dotprod39/1 -> Mux/39
  "IW{1,1}(40,:)'"/1 -> dotprod40/1
  dotprod40/1 -> Mux/40
  "IW{1,1}(41,:)'"/1 -> dotprod41/1
  dotprod41/1 -> Mux/41
  "IW{1,1}(42,:)'"/1 -> dotprod42/1
  dotprod42/1 -> Mux/42
  "IW{1,1}(43,:)'"/1 -> dotprod43/1
  dotprod43/1 -> Mux/43
  "IW{1,1}(44,:)'"/1 -> dotprod44/1
  dotprod44/1 -> Mux/44
  "IW{1,1}(45,:)'"/1 -> dotprod45/1
  dotprod45/1 -> Mux/45
  "IW{1,1}(46,:)'"/1 -> dotprod46/1
  dotprod46/1 -> Mux/46
  "IW{1,1}(47,:)'"/1 -> dotprod47/1
  dotprod47/1 -> Mux/47
  "IW{1,1}(48,:)'"/1 -> dotprod48/1
  dotprod48/1 -> Mux/48
  "IW{1,1}(49,:)'"/1 -> dotprod49/1
  dotprod49/1 -> Mux/49
  "IW{1,1}(50,:)'"/1 -> dotprod50/1
  dotprod50/1 -> Mux/50
  Mux/1 -> "iz{1,1}"/1

== system Quadrotor_two_blocks_v3/NN/Layer 2/Delays 1 ==
  "p{2}" : Inport  PortDimensions=50
      mask Display: e = 0.06;c1 = [120 230 180]/255;c2 = ([120 230 180]+0)/(256+128);c3 = ([120 230 180]+128)/(256+128);patch([0 1 1 0],[0 0 1 1],c1);patch([0 1 1 1-e 1-e 0+e],[0 0 1 1-e 0+e 0+e],c2);patch([0 0 1 1-e 0+e 0+e],[0 1 1 1-e 1-e 0+e],c3);plot([0 1 1 0 0],[0 0 1 1 0]);
  mux : Mux  Inputs=1
      mask Display: e = 0.06;c1 = [120 150 230]/255;c2 = ([120 150 230]+0)/383;c3 = ([120 150 230]+128)/383;patch([0 1 1 0],[0 0 1 1],c1);patch([0 1 1 1-e 1-e 0+e],[0 0 1 1-e 0+e 0+e],c2);patch([0 0 1 1-e 0+e 0+e],[0 1 1 1-e 1-e 0+e],c3);plot([0 1 1 0 0],[0 0 1 1 0]);disp('Mux')
  "pd{2,1}" : Outport
      mask Display: e = 0.06;c1 = [120 230 180]/255;c2 = ([120 230 180]+0)/(256+128);c3 = ([120 230 180]+128)/(256+128);patch([0 1 1 0],[0 0 1 1],c1);patch([0 1 1 1-e 1-e 0+e],[0 0 1 1-e 0+e 0+e],c2);patch([0 0 1 1-e 0+e 0+e],[0 1 1 1-e 1-e 0+e],c3);plot([0 1 1 0 0],[0 0 1 1 0]);
  wires:
  "p{2}"/1 -> mux/1
  mux/1 -> "pd{2,1}"/1
